simulink model "Lab3PartB"  (R2013b)
settings: Solver=ode45  StartTime=0.0  StopTime=15.5  RelTol=1e-3
libraries: simulink x1
settings Model: Creator=Kalai  LastModifiedBy=Kalai

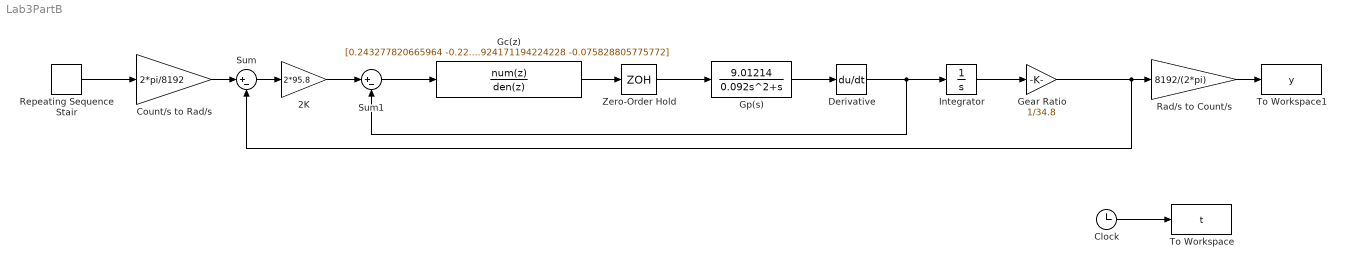
== system Lab3PartB ==
  2K : Gain  Gain=2*95.8
  Clock : Clock
  Count/s to Rad/s : Gain  Gain=2*pi/8192
  Derivative : Derivative
  Gc(z) : DiscreteTransferFcn  Numerator=[0.243277820665964 -0.226212950046755 0]  Denominator=[1 -0.924171194224228 -0.075828805775772]  SampleTime=0.008
  Gear Ratio : Gain  Gain=1/34.8
  Gp(s) : TransferFcn  Numerator=[9.01214]  Denominator=[0.092 1 0]
  Integrator : Integrator
  Rad/s to Count/s : Gain  Gain=8192/(2*pi)
  Repeating Sequence Stair : simulink/Sources/Repeating Sequence Stair  OutValues=|  tsamp=-1  OutMin=[]  OutMax=[]  OutDataTypeStr=double  OutputDataTypeScalingMode=double  OutDataType=fixdt(0,8)  ConRadixGroup=Best Precision: Vector-wise  OutScaling=2^-12
      | [3072
      | 3072
      | 3072
      | 3072
      | 3072
      | 3072
      | 3072
      | 3072
      | 3072
      | 3072
      | 3072
      | 3072
      | 3072
      | 3072
      | 3072
      | 3072
      | 3072
      | 3072
      | 3072
      | 3072
      | 3072
      | 3072
      | 3072
      | 3072
      | 3072
      | 3072
      | 3072
      | 3072
      | 3072
      | 3072
      | 3072
      | 3072
      | 3072
      | 3072
      | 3072
      | 3072
      | 3072
      | 3072
      | 3072
      | 3072
      | 3072
      | 3072
      | 3072
      | 3072
      | 3072
      | 3072
      | 3072
      | 3072
      | 3072
      | 3072
      | 3072
      | 3072
      | 3072
      | 3072
      | 3072
      | 3072
      | 3072
      | 3072
      | 3072
      | 3072
      | 3072
      | 3072
      | 3072
      | 3072
      | 3072
      | 3072
      | 3072
      | 3072
      | 3072
      | 3072
      | 3072
      | 3072
      | 3072
      | 3072
      | 3072
      | 3072
      | 3072
      | 3072
      | 3072
      | 3072
      | 3072
      | 3072
      | 3072
      | 3072
      | 3072
      | 3072
      | 3072
      | 3072
      | 3072
      | 3072
      | 3072
      | 3072
      | 3072
      | 3072
      | 3072
      | 3072
      | 3072
      | 3072
      | 3072
      | 3072
      | 3072
      | 3072
      | 3072
      | 3072
      | 3072
      | 3072
      | 3072
      | 3072
      | 3072
      | 3072
      | 3072
      | 3072
      | 3072
      | 3072
      | 3072
      | 3072
      | 3072
      | 3072
      | 3072
      | 3072
      | 3072
      | 3072
      | 3072
      | 3072
      | 3072
      | 3072
      | 3072
      | 3072
      | 3072
      | 3072
      | 3072
      | 3072
      | 3072
      | 3072
      | 3072
      | 3072
      | 3072
      | 3072
      | 3072
      | 3072
      | 3072
      | 3072
      | 3072
      | 3072
      | 3072
      | 3072
      | 3072
      | 3072
      | 3072
      | 3072
      | 3072
      | 3072
      | 3072
      | 3072
      | 3072
      | 3072
      | 3072
      | 3072
      | 3072
      | 3072
      | 3072
      | 3072
      | 3072
      | 3072
      | 3072
      | 3072
      | 3072
      | 3072
      | 3072
      | 3072
      | 3072
      | 3072
      | 3072
      | 3072
      | 3072
      | 3072
      | 3072
      | 3072
      | 3072
      | 3072
      | 3072
      | 3072
      | 3072
      | 3072
      | 3072
      | 3072
      | 3072
      | 3072
      | 3072
      | 3072
      | 3072
      | 3072
      | 3072
      | 3072
      | 3072
      | 3072
      | 3072
      | 3072
      | 3072
      | 3072
      | 3072
      | 3072
      | 3072
      | 3072
      | 3072
      | 3072
      | 3072
      | 3072
      | 3072
      | 3072
      | 3072
      | 3072
      | 3072
      | 3072
      | 3072
      | 3072
      | 3072
      | 3072
      | 3072
      | 3072
      | 3072
      | 3072
      | 3072
      | 3072
      | 3072
      | 3072
      | 3072
      | 3072
      | 3072
      | 3072
      | 3072
      | 3072
      | 3072
      | 3072
      | 3072
      | 3072
      | 3072
      | 3072
      | 3072
      | 3072
      | 3072
      | 3072
      | 3072
      | 3072
      | 3072
      | 3072
      | 3072
      | 3072
      | 3072
      | 3072
      | 3072
      | 3072
      | 3072
      | 3072
      | 3072
      | 3072
      | 3072
      | 3072
      | 3072
      | 3072
      | 3072
      | 3072
      | 3072
      | 3072
      | 3072
      | 3072
      | 3072
      | 3072
      | 3072
      | 3072
      | 3072
      | 3072
      | 3072
      | 3072
      | 3072
      | 3072
      | 3072
      | 3072
      | 3072
      | 3072
      | 3072
      | 3072
      | 3072
      | 3072
      | 3072
      | 3072
      | 3072
      | 3072
      | 3072
      | 3072
      | 3072
      | 3072
      | 3072
      | 3072
      | 3072
      | 3072
      | 3072
      | 3072
      | 3072
      | 3072
      | 3072
      | 3072
      | 3072
      | 3072
      | 3072
      | 3072
      | 3072
      | 3072
      | 3072
      | 3072
      | 3072
      | 3072
      | 3072
      | 3072
      | 3072
      | 3072
      | 3072
      | 3072
      | 3072
      | 3072
      | 3072
      | 3072
      | 3072
      | 3072
      | 3072
      | 3072
      | 3072
      | 3072
      | 3072
      | 3072
      | 3072
      | 3072
      | 3072
      | 3072
      | 3072
      | 3072
      | 3072
      | 3072
      | 3072
      | 3072
      | 3072
      | 3072
      | 3072
      | 3072
      | 3072
      | 3072
      | 3072
      | 3072
      | 3072
      | 3072
      | 3072
      | 3072
      | 3072
      | 3072
      | 3072
      | 3072
      | 3072
      | 3072
      | 3072
      | 3072
      | 3072
      | 3072
      | 3072
      | 3072
      | 3072
      | 3072
      | 3072
      | 3072
      | 3072
      | 3072
      | 3072
      | 3072
      | 3072
      | 3072
      | 3072
      | 3072
      | 3072
      | 3072
      | 3072
      | 3072
      | 3072
      | 3072
      | 3072
      | 3072
      | 3072
      | 3072
      | 3072
      | 3072
      | 3072
      | 3072
      | 3072
      | 3072
      | 3072
      | 3072
      | 3072
      | 3072
      | 3072
      | 3072
      | 3072
      | 3072
      | 1024
      | 1024
      | 1024
      | 1024
      | 1024
      | 1024
      | 1024
      | 1024
      | 1024
      | 1024
      | 1024
      | 1024
      | 1024
      | 1024
      | 1024
      | 1024
      | 1024
      | 1024
      | 1024
      | 1024
      | 1024
      | 1024
      | 1024
      | 1024
      | 1024
      | 1024
      | 1024
      | 1024
      | 1024
      | 1024
      | 1024
      | 1024
      | 1024
      | 1024
      | 1024
      | 1024
      | 1024
      | 1024
      | 1024
      | 1024
      | 1024
      | 1024
      | 1024
      | 1024
      | 1024
      | 1024
      | 1024
      | 1024
      | 1024
      | 1024
      | 1024
      | 1024
      | 1024
      | 1024
      | 1024
      | 1024
      | 1024
      | 1024
      | 1024
      | 1024
      | 1024
      | 1024
      | 1024
      | 1024
      | 1024
      | 1024
      | 1024
      | 1024
      | 1024
      | 1024
      | 1024
      | 1024
      | 1024
      | 1024
      | 1024
      | 1024
      | 1024
      | 1024
      | 1024
      | 1024
      | 1024
      | 1024
      | 1024
      | 1024
      | 1024
      | 1024
      | 1024
      | 1024
      | 1024
      | 1024
      | 1024
      | 1024
      | 1024
      | 1024
      | 1024
      | 1024
      | 1024
      | 1024
      | 1024
      | 1024
      | 1024
      | 1024
      | 1024
      | 1024
      | 1024
      | 1024
      | 1024
      | 1024
      | 1024
      | 1024
      | 1024
      | 1024
      | 1024
      | 1024
      | 1024
      | 1024
      | 1024
      | 1024
      | 1024
      | 1024
      | 1024
      | 1024
      | 1024
      | 1024
      | 1024
      | 1024
      | 1024
      | 1024
      | 1024
      | 1024
      | 1024
      | 1024
      | 1024
      | 1024
      | 1024
      | 1024
      | 1024
      | 1024
      | 1024
      | 1024
      | 1024
      | 1024
      | 1024
      | 1024
      | 1024
      | 1024
      | 1024
      | 1024
      | 1024
      | 1024
      | 1024
      | 1024
      | 1024
      | 1024
      | 1024
      | 1024
      | 1024
      | 1024
      | 1024
      | 1024
      | 1024
      | 1024
      | 1024
      | 1024
      | 1024
      | 1024
      | 1024
      | 1024
      | 1024
      | 1024
      | 1024
      | 1024
      | 1024
      | 1024
      | 1024
      | 1024
      | 1024
      | 1024
      | 1024
      | 1024
      | 1024
      | 1024
      | 1024
      | 1024
      | 1024
      | 1024
      | 1024
      | 1024
      | 1024
      | 1024
      | 1024
      | 1024
      | 1024
      | 1024
      | 1024
      | 1024
      | 1024
      | 1024
      | 1024
      | 1024
      | 1024
      | 1024
      | 1024
      | 1024
      | 1024
      | 1024
      | 1024
      | 1024
      | 1024
      | 1024
      | 1024
      | 1024
      | 1024
      | 1024
      | 1024
      | 1024
      | 1024
      | 1024
      | 1024
      | 1024
      | 1024
      | 1024
      | 1024
      | 1024
      | 1024
      | 1024
      | 1024
      | 1024
      | 1024
      | 1024
      | 1024
      | 1024
      | 1024
      | 1024
      | 1024
      | 1024
      | 1024
      | 1024
      | 1024
      | 1024
      | 1024
      | 1024
      | 1024
      | 1024
      | 1024
      | 1024
      | 1024
      | 1024
      | 1024
      | 1024
      | 1024
      | 1024
      | 1024
      | 1024
      | 1024
      | 1024
      | 1024
      | 1024
      | 1024
      | 1024
      | 1024
      | 1024
      | 1024
      | 1024
      | 1024
      | 1024
      | 1024
      | 1024
      | 1024
      | 1024
      | 1024
      | 1024
      | 1024
      | 1024
      | 1024
      | 1024
      | 1024
      | 1024
      | 1024
      | 1024
      | 1024
      | 1024
      | 1024
      | 1024
      | 1024
      | 1024
      | 1024
      | 1024
      | 1024
      | 1024
      | 1024
      | 1024
      | 1024
      | 1024
      | 1024
      | 1024
      | 1024
      | 1024
      | 1024
      | 1024
      | 1024
      | 1024
      | 1024
      | 1024
      | 1024
      | 1024
      | 1024
      | 1024
      | 1024
      | 1024
      | 1024
      | 1024
      | 1024
      | 1024
      | 1024
      | 1024
      | 1024
      | 1024
      | 1024
      | 1024
      | 1024
      | 1024
      | 1024
      | 1024
      | 1024
      | 1024
      | 1024
      | 1024
      | 1024
      | 1024
      | 1024
      | 1024
      | 1024
      | 1024
      | 1024
      | 1024
      | 1024
      | 1024
      | 1024
      | 1024
      | 1024
      | 1024
      | 1024
      | 1024
      | 1024
      | 1024
      | 1024
      | 1024
      | 1024
      | 1024
      | 1024
      | 1024
      | 1024
      | 1024
      | 1024
      | 1024
      | 1024
      | 1024
      | 1024
      | 1024
      | 1024
      | 1024
      | 1024
      | 1024
      | 1024
      | 1024
      | 1024
      | 1024
      | 1024
      | 1024
      | 1024
      | 1024
      | 1024
      | 1024
      | 1024
      | 1024
      | 1024
      | 1024
      | 1024
      | 1024
      | 1024
      | 1024
      | 1024
      | 1024
      | 1024
      | 1024
      | 1024
      | 1024
      | 1024
      | 1024
      | 1024
      | 1024
      | 1024
      | 1024
      | 1024
      | 1024
      | 1024
      | 1024
      | 1024
      | 1024
      | 2048
      | 2048
      | 2048
      | 2048
      | 2048
      | 2048
      | 2048
      | 2048
      | 2048
      | 2048
      | 2048
      | 2048
      | 2048
      | 2048
      | 2048
      | 2048
      | 2048
      | 2048
      | 2048
      | 2048
      | 2048
      | 2048
      | 2048
      | 2048
      | 2048
      | 2048
      | 2048
      | 2048
      | 2048
      | 2048
      | 2048
      | 2048
      | 2048
      | 2048
      | 2048
      | 2048
      | 2048
      | 2048
      | 2048
      | 2048
      | 2048
      | 2048
      | 2048
      | 2048
      | 2048
      | 2048
      | 2048
      | 2048
      | 2048
      | 2048
      | 2048
      | 2048
      | 2048
      | 2048
      | 2048
      | 2048
      | 2048
      | 2048
      | 2048
      | 2048
      | 2048
      | 2048
      | 2048
      | 2048
      | 2048
      | 2048
      | 2048
      | 2048
      | 2048
      | 2048
      | 2048
      | 2048
      | 2048
      | 2048
      | 2048
      | 2048
      | 2048
      | 2048
      | 2048
      | 2048
      | 2048
      | 2048
      | 2048
      | 2048
      | 2048
      | 2048
      | 2048
      | 2048
      | 2048
      | 2048
      | 2048
      | 2048
      | 2048
      | 2048
      | 2048
      | 2048
      | 2048
      | 2048
      | 2048
      | 2048
      | 2048
      | 2048
      | 2048
      | 2048
      | 2048
      | 2048
      | 2048
      | 2048
      | 2048
      | 2048
      | 2048
      | 2048
      | 2048
      | 2048
      | 2048
      | 2048
      | 2048
      | 2048
      | 2048
      | 2048
      | 2048
      | 2048
      | 2048
      | 2048
      | 2048
      | 2048
      | 2048
      | 2048
      | 2048
      | 2048
      | 2048
      | 2048
      | 2048
      | 2048
      | 2048
      | 2048
      | 2048
      | 2048
      | 2048
      | 2048
      | 2048
      | 2048
      | 2048
      | 2048
      | 2048
      | 2048
      | 2048
      | 2048
      | 2048
      | 2048
      | 2048
      | 2048
      | 2048
      | 2048
      | 2048
      | 2048
      | 2048
      | 2048
      | 2048
      | 2048
      | 2048
      | 2048
      | 2048
      | 2048
      | 2048
      | 2048
      | 2048
      | 2048
      | 2048
      | 2048
      | 2048
      | 2048
      | 2048
      | 2048
      | 2048
      | 2048
      | 2048
      | 2048
      | 2048
      | 2048
      | 2048
      | 2048
      | 2048
      | 2048
      | 2048
      | 2048
      | 2048
      | 2048
      | 2048
      | 2048
      | 2048
      | 2048
      | 2048
      | 2048
      | 2048
      | 2048
      | 2048
      | 2048
      | 2048
      | 2048
      | 2048
      | 2048
      | 2048
      | 2048
      | 2048
      | 2048
      | 2048
      | 2048
      | 2048
      | 2048
      | 2048
      | 2048
      | 2048
      | 2048
      | 2048
      | 2048
      | 2048
      | 2048
      | 2048
      | 2048
      | 2048
      | 2048
      | 2048
      | 2048
      | 2048
      | 2048
      | 2048
      | 2048
      | 2048
      | 2048
      | 2048
      | 2048
      | 2048
      | 2048
      | 2048
      | 2048
      | 2048
      | 2048
      | 2048
      | 2048
      | 2048
      | 2048
      | 2048
      | 2048
      | 2048
      | 2048
      | 2048
      | 2048
      | 2048
      | 2048
      | 2048
      | 2048
      | 2048
      | 2048
      | 2048
      | 2048
      | 2048
      | 2048
      | 2048
      | 2048
      | 2048
      | 2048
      | 2048
      | 2048
      | 2048
      | 2048
      | 2048
      | 2048
      | 2048
      | 2048
      | 2048
      | 2048
      | 2048
      | 2048
      | 2048
      | 2048
      | 2048
      | 2048
      | 2048
      | 2048
      | 2048
      | 2048
      | 2048
      | 2048
      | 2048
      | 2048
      | 2048
      | 2048
      | 2048
      | 2048
      | 2048
      | 2048
      | 2048
      | 2048
      | 2048
      | 2048
      | 2048
      | 2048
      | 2048
      | 2048
      | 2048
      | 2048
      | 2048
      | 2048
      | 2048
      | 2048
      | 2048
      | 2048
      | 2048
      | 2048
      | 2048
      | 2048
      | 2048
      | 2048
      | 2048
      | 2048
      | 2048
      | 2048
      | 2048
      | 2048
      | 2048
      | 2048
      | 2048
      | 2048
      | 2048
      | 2048
      | 2048
      | 2048
      | 2048
      | 2048
      | 2048
      | 2048
      | 2048
      | 2048
      | 2048
      | 2048
      | 2048
      | 2048
      | 2048
      | 2048
      | 2048
      | 2048
      | 2048
      | 2048
      | 2048
      | 2048
      | 2048
      | 2048
      | 2048
      | 2048
      | 2048
      | 2048
      | 2048
      | 2048
      | 2048
      | 2048
      | 2048
      | 2048
      | 2048
      | 2048
      | 2048
      | 2048
      | 2048
      | 2048
      | 2048
      | 2048
      | 2048
      | 2048
      | 2048
      | 2048
      | 2048
      | 2048
      | 2048
      | 2048
      | 2048
      | 2048
      | 2048
      | 2048
      | 2048
      | 2048
      | 2048
      | 2048
      | 2048
      | 2048
      | 2048
      | 2048
      | 2048
      | 2048
      | 2048
      | 2048
      | 2048
      | 2048
      | 2048
      | 2048
      | 2048
      | 2048
      | 2048
      | 2048
      | 2048
      | 2048
      | 2560
      | 2560
      | 2560
      | 2560
      | 2560
      | 2560
      | 2560
      | 2560
      | 2560
      | 2560
      | 2560
      | 2560
      | 2560
      | 2560
      | 2560
      | 2560
      | 2560
      | 2560
      | 2560
      | 2560
      | 2560
      | 2560
      | 2560
      | 2560
      | 2560
      | 2560
      | 2560
      | 2560
      | 2560
      | 2560
      | 2560
      | 2560
      | 2560
      | 2560
      | 2560
      | 2560
      | 2560
      | 2560
      | 2560
      | 2560
      | 2560
      | 2560
      | 2560
      | 2560
      | 2560
      | 2560
      | 2560
      | 2560
      | 2560
      | 2560
      | 2560
      | 2560
      | 2560
      | 2560
      | 2560
      | 2560
      | 2560
      | 2560
      | 2560
      | 2560
      | 2560
      | 2560
      | 2560
      | 2560
      | 2560
      | 2560
      | 2560
      | 2560
      | 2560
      | 2560
      | 2560
      | 2560
      | 2560
      | 2560
      | 2560
      | 2560
      | 2560
      | 2560
      | 2560
      | 2560
      | 2560
      | 2560
      | 2560
      | 2560
      | 2560
      | 2560
      | 2560
      | 2560
      | 2560
      | 2560
      | 2560
      | 2560
      | 2560
      | 2560
      | 2560
      | 2560
      | 2560
      | 2560
      | 2560
      | 2560
      | 2560
      | 2560
      | 2560
      | 2560
      | 2560
      | 2560
      | 2560
      | 2560
      | 2560
      | 2560
      | 2560
      | 2560
      | 2560
      | 2560
      | 2560
      | 2560
      | 2560
      | 2560
      | 2560
      | 2560
      | 2560
      | 2560
      | 2560
      | 2560
      | 2560
      | 2560
      | 2560
      | 2560
      | 2560
      | 2560
      | 2560
      | 2560
      | 2560
      | 2560
      | 2560
      | 2560
      | 2560
      | 2560
      | 2560
      | 2560
      | 2560
      | 2560
      | 2560
      | 2560
      | 2560
      | 2560
      | 2560
      | 2560
      | 2560
      | 2560
      | 2560
      | 2560
      | 2560
      | 2560
      | 2560
      | 2560
      | 2560
      | 2560
      | 2560
      | 2560
      | 2560
      | 2560
      | 2560
      | 2560
      | 2560
      | 2560
      | 2560
      | 2560
      | 2560
      | 2560
      | 2560
      | 2560
      | 2560
      | 2560
      | 2560
      | 2560
      | 2560
      | 2560
      | 2560
      | 2560
      | 2560
      | 2560
      | 2560
      | 2560
      | 2560
      | 2560
      | 2560
      | 2560
      | 2560
      | 2560
      | 2560
      | 2560
      | 2560
      | 2560
      | 2560
      | 2560
      | 2560
      | 2560
      | 2560
      | 2560
      | 2560
      | 2560
      | 2560
      | 2560
      | 2560
      | 2560
      | 2560
      | 2560
      | 2560
      | 2560
      | 2560
      | 2560
      | 2560
      | 2560
      | 2560
      | 2560
      | 2560
      | 2560
      | 2560
      | 2560
      | 2560
      | 2560
      | 2560
      | 2560
      | 2560
      | 2560
      | 2560
      | 2560
      | 2560
      | 2560
      | 2560
      | 2560
      | 2560
      | 2560
      | 2560
      | 2560
      | 2560
      | 2560
      | 2560
      | 2560
      | 2560
      | 2560
      | 2560
      | 2560
      | 2560
      | 2560
      | 2560
      | 2560
      | 2560
      | 2560
      | 2560
      | 2560
      | 2560
      | 2560
      | 2560
      | 2560
      | 2560
      | 2560
      | 2560
      | 2560
      | 2560
      | 2560
      | 2560
      | 2560
      | 2560
      | 2560
      | 2560
      | 2560
      | 2560
      | 2560
      | 2560
      | 2560
      | 2560
      | 2560
      | 2560
      | 2560
      | 2560
      | 2560
      | 2560
      | 2560
      | 2560
      | 2560
      | 2560
      | 2560
      | 2560
      | 2560
      | 2560
      | 2560
      | 2560
      | 2560
      | 2560
      | 2560
      | 2560
      | 2560
      | 2560
      | 2560
      | 2560
      | 2560
      | 2560
      | 2560
      | 2560
      | 2560
      | 2560
      | 2560
      | 2560
      | 2560
      | 2560
      | 2560
      | 2560
      | 2560
      | 2560
      | 2560
      | 2560
      | 2560
      | 2560
      | 2560
      | 2560
      | 2560
      | 2560
      | 2560
      | 2560
      | 2560
      | 2560
      | 2560
      | 2560
      | 2560
      | 2560
      | 2560
      | 2560
      | 2560
      | 2560
      | 2560
      | 2560
      | 2560
      | 2560
      | 2560
      | 2560
      | 2560
      | 2560
      | 2560
      | 2560
      | 2560
      | 2560
      | 2560
      | 2560
      | 2560
      | 2560
      | 2560
      | 2560
      | 2560
      | 2560
      | 2560
      | 2560
      | 2560
      | 2560
      | 2560
      | 2560
      | 2560
      | 2560
      | 2560
      | 2560
      | 2560
      | 2560
      | 2560
      | 2560
      | 2560
      | 2560
      | 2560
      | 2560
      | 2560
      | 2560
      | 2560
      | 2560
      | 2560
      | 2560
      | 2560
      | 2560
      | 2560
      | 2560
      | 2560
      | 2560
      | 2560
      | 2560
      | 2560
      | 2560
      | 2560
      | 2560
      | 2560
      | 2560
      | 2560
      | 2560
      | 2560
      | 2560
      | 2560
      | 2560
      | 2560
      | 2560
      | 2560
      | 2560
      | 2560
      | 0
      | 0
      | 0
      | 0
      | 0
      | 0
      | 0
      | 0
      | 0
      | 0
      | 0
      | 0
      | 0
      | 0
      | 0
      | 0
      | 0
      | 0
      | 0
      | 0
      | 0
      | 0
      | 0
      | 0
      | 0
      | 0
      | 0
      | 0
      | 0
      | 0
      | 0
      | 0
      | 0
      | 0
      | 0
      | 0
      | 0
      | 0
      | 0
      | 0
      | 0
      | 0
      | 0
      | 0
      | 0
      | 0
      | 0
      | 0
      | 0
      | 0
      | 0
      | 0
      | 0
      | 0
      | 0
      | 0
      | 0
      | 0
      | 0
      | 0
      | 0
      | 0
      | 0
      | 0
      | 0
      | 0
      | 0
      | 0
      | 0
      | 0
      | 0
      | 0
      | 0
      | 0
      | 0
      | 0
      | 0
      | 0
      | 0
      | 0
      | 0
      | 0
      | 0
      | 0
      | 0
      | 0
      | 0
      | 0
      | 0
      | 0
      | 0
      | 0
      | 0
      | 0
      | 0
      | 0
      | 0
      | 0
      | 0
      | 0
      | 0
      | 0
      | 0
      | 0
      | 0
      | 0
      | 0
      | 0
      | 0
      | 0
      | 0
      | 0
      | 0
      | 0
      | 0
      | 0
      | 0
      | 0
      | 0
      | 0
      | 0
      | 0
      | 0
      | 0
      | 0
      | 0
      | 0
      | 0
      | 0
      | 0
      | 0
      | 0
      | 0
      | 0
      | 0
      | 0
      | 0
      | 0
      | 0
      | 0
      | 0
      | 0
      | 0
      | 0
      | 0
      | 0
      | 0
      | 0
      | 0
      | 0
      | 0
      | 0
      | 0
      | 0
      | 0
      | 0
      | 0
      | 0
      | 0
      | 0
      | 0
      | 0
      | 0
      | 0
      | 0
      | 0
      | 0
      | 0
      | 0
      | 0
      | 0
      | 0
      | 0
      | 0
      | 0
      | 0
      | 0
      | 0
      | 0
      | 0
      | 0
      | 0
      | 0
      | 0
      | 0
      | 0
      | 0
      | 0
      | 0
      | 0
      | 0
      | 0
      | 0
      | 0
      | 0
      | 0
      | 0
      | 0
      | 0
      | 0
      | 0
      | 0
      | 0
      | 0
      | 0
      | 0
      | 0
      | 0
      | 0
      | 0
      | 0
      | 0
      | 0
      | 0
      | 0
      | 0
      | 0
      | 0
      | 0
      | 0
      | 0
      | 0
      | 0
      | 0
      | 0
      | 0
      | 0
      | 0
      | 0
      | 0
      | 0
      | 0
      | 0
      | 0
      | 0
      | 0
      | 0
      | 0
      | 0
      | 0
      | 0
      | 0
      | 0
      | 0
      | 0
      | 0
      | 0
      | 0
      | 0
      | 0
      | 0
      | 0
      | 0
      | 0
      | 0
      | 0
      | 0
      | 0
      | 0
      | 0
      | 0
      | 0
      | 0
      | 0
      | 0
      | 0
      | 0
      | 0
      | 0
      | 0
      | 0
      | 0
      | 0
      | 0
      | 0
      | 0
      | 0
      | 0
      | 0
      | 0
      | 0
      | 0
      | 0
      | 0
      | 0
      | 0
      | 0
      | 0
      | 0
      | 0
      | 0
      | 0
      | 0
      | 0
      | 0
      | 0
      | 0
      | 0
      | 0
      | 0
      | 0
      | 0
      | 0
      | 0
      | 0
      | 0
      | 0
      | 0
      | 0
      | 0
      | 0
      | 0
      | 0
      | 0
      | 0
      | 0
      | 0
      | 0
      | 0
      | 0
      | 0
      | 0
      | 0
      | 0
      | 0
      | 0
      | 0
      | 0
      | 0
      | 0
      | 0
      | 0
      | 0
      | 0
      | 0
      | 0
      | 0
      | 0
      | 0
      | 0
      | 0
      | 0
      | 0
      | 0
      | 0
      | 0
      | 0
      | 0
      | 0
      | 0
      | 0
      | 0
      | 0
      | 0
      | 0
      | 0
      | 0
      | 0
      | 0
      | 0
      | 0
      | 0
      | 0
      | 0
      | 0
      | 0
      | 0
      | 0
      | 0
      | 0
      | 0
      | 0
      | 0
      | 0
      | 0
      | 0
      | 0
      | 0
      | 0
      | 0
      | 0
      | 0
      | 0
      | 0
      | 0
      | 0
      | 0
      | 0
      | 0
      | 0
      | 0
      | 0
      | 0
      | 0
      | 0
      | 0
      | 0
      | 0
      | 0
      | 0].'
  Sum : Sum  Inputs=|+-
  Sum1 : Sum  Inputs=|+-
  To Workspace : ToWorkspace  VariableName=t  SampleTime=-1
  To Workspace1 : ToWorkspace  VariableName=y  SampleTime=-1
  Zero-Order Hold : ZeroOrderHold  SampleTime=0.008
  wires:
  Sum/1 -> 2K/1
  Count/s to Rad/s/1 -> Sum/1
  2K/1 -> Sum1/1
  Sum1/1 -> Gc(z)/1
  Gc(z)/1 -> Zero-Order Hold/1
  Zero-Order Hold/1 -> Gp(s)/1
  Gp(s)/1 -> Derivative/1
  Derivative/1 -> Sum1/2, Integrator/1
  Integrator/1 -> Gear Ratio/1
  Gear Ratio/1 -> Sum/2, Rad/s to Count/s/1
  Rad/s to Count/s/1 -> To Workspace1/1
  Clock/1 -> To Workspace/1
  Repeating Sequence Stair/1 -> Count/s to Rad/s/1
